simulink model "sldemo_interp_memory_org"  (Simulink 10.0)
settings: Solver=FixedStepDiscrete  StartTime=0.0  StopTime=10.0  FixedStep=1  RelTol=1e-3  EnableMultiTasking=on
Description:
  | Saving Memory in Prelookup and Interpolation Blocks by Using Smaller Data
  | This example shows how to save memory in Prelookup and Interpolation blocks.
  | The Prelookup and Interpolation Using Prelookup blocks allow the data type storing breakpoints
  | and table data to be set explicitly. Note that the Prelookup block allows the breakpoint data to differ
  | from the input data type, and the Interpolation Using Prelookup block allows the table data to
  | differ from the output data type.
  | 
  | In this model, the breakpoints and table are stored using single precision floating-point data type,
  | and the calculations are performed using double precision floating-point data type. This reduces
  | the amount of breakpoint and table data memory by half.
  | 
  | To see this in the generated code, open the model and build it.
settings Model: Creator=The MathWorks, Inc.  LastModifiedBy=bhisma
settings DataIOCC: LimitDataPoints=on  SaveFormat=StructureWithTime  ReturnWorkspaceOutputs=on
settings OptimizationCC: DefaultParameterBehavior=Inlined  ExpressionDepthLimit=2147483647
settings DebuggingCC: UnderspecifiedInitializationDetection=Simplified  MergeDetectMultiDrivingBlocksExec=error  SolverPrmCheckMsg=warning  ParameterPrecisionLossMsg=none  FcnCallInpInsideContextMsg=warning  StateNameClashWarn=warning
settings HardwareCC: TargetHWDeviceType=32-bit Generic
settings RTWCC: GenCodeOnly=on  GenerateReport=on  RTWVerbose=off  LaunchReport=on
settings GRTTargetCC: GeneratePreprocessorConditionals=Disable all
settings ConfigComp: CovExternalEMLEnable=off

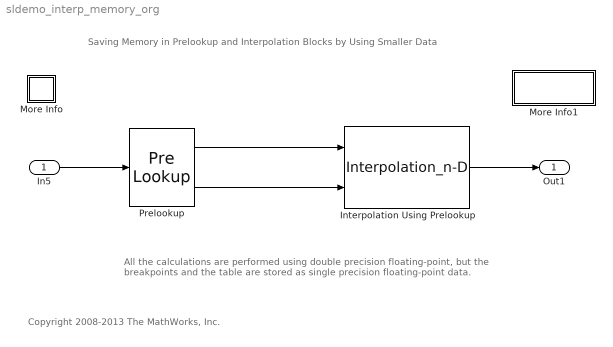
== system sldemo_interp_memory_org ==
  note: Copyright 2008-2013 The MathWorks, Inc.
  note: All the calculations are performed using double precision floating-point,
      | but the breakpoints and the table are stored as single precision floating-point data.
  note: Saving Memory in Prelookup and Interpolation Blocks by Using Smaller Data
  In5 : Inport  OutDataTypeStr=double
  Interpolation Using Prelookup : Interpolation_n-D  NumberOfTableDimensions=1  Table=sin(linspace(0,pi/4,11))  ExtrapMethod=Clip  RemoveProtectionIndex=on  OutDataTypeStr=double  TableDataTypeStr=single
      settings: AttributesFormatString=Table type = %<TableDataTypeStr>  InputPortMap=u0,u1
  More Info : Subsystem
      settings: OpenFcn=showdemo(bdroot(gcs))
      mask Display: disp('?')
  More Info1 : Subsystem
      settings: OpenFcn=rtwbuild(bdroot(gcs))
      mask Display: fprintf('Double-click to\ngenerate code')
  Prelookup : PreLookup  BreakpointsData=exp(linspace(1,3,11))  BreakpointDataTypeStr=single  FractionDataTypeStr=double
      settings: AttributesFormatString=Breakpoint type = %<BreakpointDataTypeStr>
  Out1 : Outport  VectorParamsAs1DForOutWhenUnconnected=off
  wires:
  Interpolation Using Prelookup/1 -> Out1/1
  In5/1 -> Prelookup/1
  Prelookup/1 -> Interpolation Using Prelookup/1
  Prelookup/2 -> Interpolation Using Prelookup/2

== system sldemo_interp_memory_org/More Info ==

== system sldemo_interp_memory_org/More Info1 ==
